simulink library "outp"  (R2021b)
(part 3 of 10)

  bus_selector16/53 -> outpmodule/942(VVMC_ADASLDWSta_enum)  "<VVMC_ADASLDWSta_enum>"
  outpmodule/395(VOUTP_OBC4PreDTC_raw32) -> bus_creator/395
  outpmodule/345(VOUTP_HMIKey7FuncSta_enum) -> bus_creator/345
  outpmodule/919(VOUTP_LKATOIFault_flg) -> bus_creator/919
  outpmodule/560(VOUTP_DCDCEnaReq_flg) -> bus_creator/560
  outpmodule/917(VOUTP_ADASLKASta_enum) -> bus_creator/917
  bus_selector4/61 -> outpmodule/420(VDDM_DiagFRTSDTC_raw32)  "<VDDM_DiagFRTSDTC_raw32>"
  outpmodule/576(VOUTP_PwrDownReq_enum) -> bus_creator/576
  outpmodule/621(VOUTP_Change1_cnt) -> bus_creator/621
  outpmodule/622(VOUTP_Change2_cnt) -> bus_creator/622
  bus_selector2/83 -> outpmodule/86(VAPM_RRPulseCountTimeOut_flg)  "<VAPM_RRPulseCountTimeOut_flg>"
  outpmodule/624(VOUTP_SHA1_cnt) -> bus_creator/624
  outpmodule/187(VOUTP_DrDoorSW_flg) -> bus_creator/187
  outpmodule/990(VOUTP_CAASActive_flg) -> bus_creator/990
  outpmodule/623(VOUTP_Dash2_cnt) -> bus_creator/623
  outpmodule/620(VOUTP_Dash1_cnt) -> bus_creator/620
  outpmodule/783(VOUTP_RRP20_raw8) -> bus_creator/783
  outpmodule/618(VOUTP_Country2_cnt) -> bus_creator/618
  outpmodule/234(VOUTP_AmbLightBrightness3_enum) -> bus_creator/234
  outpmodule/509(VOUTP_CAN1BusErrorDTC_raw32) -> bus_creator/509
  bus_selector2/34 -> outpmodule/37(VAPM_USSStaFLR_flg)  "<VAPM_USSStaFLR_flg>"
  outpmodule/619(VOUTP_Variation_cnt) -> bus_creator/619
  outpmodule/176(VOUTP_RAPSErrWarnSta_enum) -> bus_creator/176
  outpmodule/617(VOUTP_Country1_cnt) -> bus_creator/617
  outpmodule/616(VOUTP_Patch2_cnt) -> bus_creator/616
  outpmodule/985(VOUTP_APSReq_enum) -> bus_creator/985
  outpmodule/613(VOUTP_Minor1_cnt) -> bus_creator/613
  bus_selector3/164 -> outpmodule/342(VBCM_HMIKey4FuncSta_enum)  "<VBCM_HMIKey4FuncSta_enum>"
  outpmodule/767(VOUTP_LFSensorMode_flg) -> bus_creator/767
  outpmodule/538(VOUTP_FDCDKCAllowSleep_flg) -> bus_creator/538
  outpmodule/615(VOUTP_Patch1_cnt) -> bus_creator/615
  bus_selector16/66 -> outpmodule/955(VVMC_ADASLaneModeR_enum)  "<VVMC_ADASLaneModeR_enum>"
  outpmodule/614(VOUTP_Minor2_cnt) -> bus_creator/614
  outpmodule/349(VOUTP_PasWdwReqAP_enum) -> bus_creator/349
  outpmodule/552(VOUTP_ActiveWU_flg) -> bus_creator/552
  outpmodule/611(VOUTP_Major1_cnt) -> bus_creator/611
  outpmodule/612(VOUTP_Major2_cnt) -> bus_creator/612
  outpmodule/335(VOUTP_AutoLockSta_flg) -> bus_creator/335
  BTHC_outputs/1 -> bus_selector11/1
  outpmodule/609(VOUTP_ECU1_cnt) -> bus_creator/609
  outpmodule/324(VOUTP_PTGUserHeight7_cnt) -> bus_creator/324
  bus_selector3/21 -> outpmodule/199(VBCM_DimmerEN_flg)  "<VBCM_DimmerEN_flg>"
  outpmodule/321(VOUTP_PTGUserHeight3_cnt) -> bus_creator/321
  outpmodule/981(VOUTP_APSActive_flg) -> bus_creator/981
  outpmodule/530(VOUTP_DKeyWelcomeSta_enum) -> bus_creator/530
  outpmodule/608(VOUTP_CarModel3_cnt) -> bus_creator/608
  outpmodule/166(VOUTP_DKCPDkeyAreaRAPSSta_enum) -> bus_creator/166
  outpmodule/606(VOUTP_CarModel1_cnt) -> bus_creator/606
  bus_selector12/75 -> outpmodule/804(VTPM_WriteChkRFID_raw)  "<VTPM_WriteChkRFID_raw>"
  bus_selector11/36 -> outpmodule/681(VTHC_sigAmbAirT_C)  "<VTHC_sigAmbAirT_C>"
  outpmodule/129(VOUTP_EPBExtReleaseAvail_flg) -> bus_creator/129
  outpmodule/607(VOUTP_CarModel2_cnt) -> bus_creator/607
  outpmodule/219(VOUTP_TrunkRel_flg) -> bus_creator/219
  outpmodule/603(VOUTP_HWVer1_cnt) -> bus_creator/603
  outpmodule/604(VOUTP_HWVer2_cnt) -> bus_creator/604
  bus_selector4/96 -> outpmodule/455(VDDM_ISAMalfuncDetDTC_raw32)  "<VDDM_ISAMalfuncDetDTC_raw32>"
  bus_selector3/39 -> outpmodule/217(VBCM_RoomLampH_flg)  "<VBCM_RoomLampH_flg>"
  outpmodule/434(VOUTP_RLRUSSDTC_raw32) -> bus_creator/434
  outpmodule/364(VOUTP_C3BMS1CSDTC_raw32) -> bus_creator/364
  outpmodule/602(VOUTP_PwrReqRAPSAvail_flg) -> bus_creator/602
  outpmodule/749(VOUTP_RRWheelDebug_flg) -> bus_creator/749
  outpmodule/556(VOUTP_PowerDownState_enum) -> bus_creator/556
  outpmodule/601(VOUTP_OTAPwrReqStdChkSta_enum) -> bus_creator/601
  outpmodule/863(VOUTP_RrUdcMax_V) -> bus_creator/863
  bus_selector11/9 -> outpmodule/654(VTHC_FDTWVCmd_pct)  "<VTHC_FDTWVCmd_pct>"
  outpmodule/932(VOUTP_ACCJerkLowerLimit_mps3) -> bus_creator/932
  outpmodule/599(VOUTP_PwrReq_OTA_enum) -> bus_creator/599
  bus_selector10/22 -> outpmodule/624(VSYS_SHA1_cnt)  "<VSYS_SHA1_cnt>"
  outpmodule/600(VOUTP_OTAPwrReqOFFChkSta_enum) -> bus_creator/600
  bus_selector6/15 -> outpmodule/535(VDKC_ParkingModeCmd_enum)  "<VDKC_ParkingModeCmd_enum>"
  outpmodule/597(VOUTP_PwrStaTOSta_enum) -> bus_creator/597
  outpmodule/390(VOUTP_MidLvSaChkDTC_raw32) -> bus_creator/390
  outpmodule/351(VOUTP_PsRWdwReqAP_enum) -> bus_creator/351
  outpmodule/459(VOUTP_MCUR1CSErrDTC_raw32) -> bus_creator/459
  outpmodule/133(VOUTP_EPBErrSta_enum) -> bus_creator/133
  outpmodule/596(VOUTP_CtrlDrPwrStbA2_flg) -> bus_creator/596
  outpmodule/329(VOUTP_TimeGapLevelSta_enum) -> bus_creator/329
  outpmodule/595(VOUTP_HWResetSta_enum) -> bus_creator/595
  outpmodule/377(VOUTP_Lv3ErrDTC_raw32) -> bus_creator/377
  outpmodule/593(VOUTP_CtrlFrBMSCCUCIR_flg) -> bus_creator/593
  outpmodule/801(VOUTP_LRPindi_enum) -> bus_creator/801
  bus_selector13/34 -> outpmodule/860(VTQD_RrIdcMin_A)  "<VTQD_RrIdcMin_A>"
  outpmodule/675(VOUTP_sigSetTempZon1St_C) -> bus_creator/675
  outpmodule/491(VOUTP_LimpHomeActTmp_flg) -> bus_creator/491
  bus_selector13/37 -> outpmodule/863(VTQD_RrUdcMax_V)  "<VTQD_RrUdcMax_V>"
  bus_selector10/30 -> outpmodule/632(VSYS_NvWriteReqRisingEdge_flg)  "<VSYS_NvWriteReqRisingEdge_flg>"
  outpmodule/782(VOUTP_LRP20_raw8) -> bus_creator/782
  outpmodule/646(VOUTP_FDCompCmd_rpm) -> bus_creator/646
  bus_selector16/102 -> outpmodule/991(VVMC_ExtraMSACtrlSta_enum)  "<VVMC_ExtraMSACtrlSta_enum>"
  outpmodule/373(VOUTP_C1ABM1CSDTC_raw32) -> bus_creator/373
  bus_selector13/35 -> outpmodule/861(VTQD_RrIdcMax_A)  "<VTQD_RrIdcMax_A>"
  bus_selector16/56 -> outpmodule/945(VVMC_ForceLowBeam_enum)  "<VVMC_ForceLowBeam_enum>"
  bus_selector13/36 -> outpmodule/862(VTQD_RrUdcMin_V)  "<VTQD_RrUdcMin_V>"
  outpmodule/226(VOUTP_AmbLightBreath1_enum) -> bus_creator/226
  outpmodule/378(VOUTP_Lv4ErrDTC_raw32) -> bus_creator/378
  bus_selector13/45 -> outpmodule/871(VTQD_ExtDoorAllow_flg)  "<VTQD_ExtDoorAllow_flg>"
  outpmodule/819(VOUTP_FlashS4ID_raw) -> bus_creator/819
  bus_selector2/91 -> outpmodule/94(VAPM_SASAngleTimeOut_flg)  "<VAPM_SASAngleTimeOut_flg>"
  bus_selector13/42 -> outpmodule/868(VTQD_DriveProtEn_flg)  "<VTQD_DriveProtEn_flg>"
  outpmodule/487(VOUTP_5vAPS1PwrErrDTC_raw32) -> bus_creator/487
  outpmodule/960(VOUTP_ADASLFCHandsOffWarning_enum) -> bus_creator/960
  bus_selector2/51 -> outpmodule/54(VAPM_RRRawWhlSpeedTimeOut_flg)  "<VAPM_RRRawWhlSpeedTimeOut_flg>"
  outpmodule/587(VOUTP_PMMAllowECUSleep_flg) -> bus_creator/587
  bus_selector13/39 -> outpmodule/865(VTQD_ExtShftAllow_flg)  "<VTQD_ExtShftAllow_flg>"
  outpmodule/951(VOUTP_LKAHODDisplayWarning_flg) -> bus_creator/951
  outpmodule/320(VOUTP_PTGUserHeight2_cnt) -> bus_creator/320
  bus_selector13/38 -> outpmodule/864(VTQD_ReBrakeLPReq_flg)  "<VTQD_ReBrakeLPReq_flg>"
  outpmodule/958(VOUTP_ADASLDWMute_flg) -> bus_creator/958
  BSYS_outputs/1 -> bus_selector10/1
  outpmodule/547(VOUTP_ErrorState_enum) -> bus_creator/547
  outpmodule/591(VOUTP_CtrlFrPwrStbA1P_flg) -> bus_creator/591
  outpmodule/203(VOUTP_RrFogLamp_flg) -> bus_creator/203
  bus_selector2/96 -> outpmodule/99(VAPM_SASCAL_flg)  "<VAPM_SASCAL_flg>"
  outpmodule/464(VOUTP_ESC1RCErrDTC_raw32) -> bus_creator/464
  bus_selector2/22 -> outpmodule/25(VAPM_PASARCL_enum)  "<VAPM_PASARCL_enum>"
  bus_selector2/19 -> outpmodule/22(VAPM_PASARMR_enum)  "<VAPM_PASARMR_enum>"
  outpmodule/999(VOUTP_FDCVMCAPSAngleTarget_deg) -> bus_creator/999
  bus_selector4/91 -> outpmodule/450(VDDM_CCUSigErrDetDTC_raw32)  "<VDDM_CCUSigErrDetDTC_raw32>"
  outpmodule/539(VOUTP_DISCTurn_flg) -> bus_creator/539
  outpmodule/169(VOUTP_CAASVMCReqA_flg) -> bus_creator/169
  bus_selector2/17 -> outpmodule/20(VAPM_APSDFLL_cm)  "<VAPM_APSDFLL_cm>"
  outpmodule/577(VOUTP_LowSOCWarn_enum) -> bus_creator/577
  bus_selector2/18 -> outpmodule/21(VAPM_PASAFCL_enum)  "<VAPM_PASAFCL_enum>"
  outpmodule/665(VOUTP_BatteryMode_enum) -> bus_creator/665
  outpmodule/1003(VOUTP_FDCVMCMaxAngCtrlOutTqLim_Nm) -> bus_creator/1003
  bus_selector2/15 -> outpmodule/18(VAPM_APSDRLL_cm)  "<VAPM_APSDRLL_cm>"
  bus_selector4/127 -> outpmodule/486(VDDM_C1EPAS2LCDTC_raw32)  "<VDDM_C1EPAS2LCDTC_raw32>"
  outpmodule/791(VOUTP_ID2messageALTU_raw8) -> bus_creator/791
  outpmodule/131(VOUTP_EPBExtApplyAvail_flg) -> bus_creator/131
  bus_selector2/10 -> outpmodule/13(VAPM_PASDFMR_cm)  "<VAPM_PASDFMR_cm>"
  bus_selector2/14 -> outpmodule/17(VAPM_APSDRLR_cm)  "<VAPM_APSDRLR_cm>"
  bus_selector2/13 -> outpmodule/16(VAPM_PASDFCL_cm)  "<VAPM_PASDFCL_cm>"
  bus_selector2/68 -> outpmodule/71(VAPM_LFPulseCountV_flg)  "<VAPM_LFPulseCountV_flg>"
  bus_selector2/89 -> outpmodule/92(VAPM_EPSAOIControlTimeOut_flg)  "<VAPM_EPSAOIControlTimeOut_flg>"
  outpmodule/947(VOUTP_ADASWarningMsg_enum) -> bus_creator/947
  bus_selector13/40 -> outpmodule/866(VTQD_CreepON_flg)  "<VTQD_CreepON_flg>"
  outpmodule/374(VOUTP_C1ABM1LCDTC_raw32) -> bus_creator/374
  bus_selector2/87 -> outpmodule/90(VAPM_DriIntendTimeOut_flg)  "<VAPM_DriIntendTimeOut_flg>"
  bus_selector2/81 -> outpmodule/84(VAPM_LRPulseCountTimeOut_flg)  "<VAPM_LRPulseCountTimeOut_flg>"
  bus_selector2/35 -> outpmodule/38(VAPM_USSStaFLL_flg)  "<VAPM_USSStaFLL_flg>"
  bus_selector2/8 -> outpmodule/11(VAPM_PASDRCR_cm)  "<VAPM_PASDRCR_cm>"
  bus_selector2/97 -> outpmodule/100(VAPM_SASCALTimeOut_flg)  "<VAPM_SASCALTimeOut_flg>"
  outpmodule/467(VOUTP_ESC5CSErrDTC_raw32) -> bus_creator/467
  outpmodule/598(VOUTP_Sched_ChgTOSta_enum) -> bus_creator/598
  bus_selector16/41 -> outpmodule/930(VVMC_ACCJerkUpperLimit_mps3)  "<VVMC_ACCJerkUpperLimit_mps3>"
  bus_selector2/9 -> outpmodule/12(VAPM_PASDRCL_cm)  "<VAPM_PASDRCL_cm>"
  bus_selector4/55 -> outpmodule/414(VDDM_ESC7NoComDTC_raw32)  "<VDDM_ESC7NoComDTC_raw32>"
  bus_selector2/6 -> outpmodule/9(VAPM_PASDRMR_cm)  "<VAPM_PASDRMR_cm>"
  bus_selector9/33 -> outpmodule/587(VPMM_PMMAllowECUSleep_flg)  "<VPMM_PMMAllowECUSleep_flg>"
  bus_selector4/116 -> outpmodule/475(VDDM_RFPressIndiDTC_raw32)  "<VDDM_RFPressIndiDTC_raw32>"
  bus_selector2/31 -> outpmodule/34(VAPM_USSStaRCL_flg)  "<VAPM_USSStaRCL_flg>"
  bus_selector13/32 -> outpmodule/858(VTQD_FrUdcMin_V)  "<VTQD_FrUdcMin_V>"
  outpmodule/772(VOUTP_S2ID_raw32) -> bus_creator/772
  bus_selector2/7 -> outpmodule/10(VAPM_PASDRML_cm)  "<VAPM_PASDRML_cm>"
  bus_selector2/5 -> outpmodule/8(VAPM_ChrgPlugSta_enum)  "<VAPM_ChrgPlugSta_enum>"
  outpmodule/455(VOUTP_ISAMalfuncDetDTC_raw32) -> bus_creator/455
  outpmodule/209(VOUTP_RBSD_flg) -> bus_creator/209
  bus_selector2/3 -> outpmodule/6(VAPM_FSOffSw_enum)  "<VAPM_FSOffSw_enum>"
  bus_selector2/2 -> outpmodule/5(VAPM_VehSpeedTimeOut_flg)  "<VAPM_VehSpeedTimeOut_flg>"
  outpmodule/642(VOUTP_DrivingMode_cnt) -> bus_creator/642
  outpmodule/380(VOUTP_BrkSWNoBacDTC_raw32) -> bus_creator/380
  outpmodule/49(VOUTP_RFRawWhlSpeed_kph) -> bus_creator/49
  bus_selector2/1 -> outpmodule/4(VAPM_VehSpeed_kph)  "<VAPM_VehSpeed_kph>"
  outpmodule/32(VOUTP_USSStaRLL_flg) -> bus_creator/32
  bus_selector2/4 -> outpmodule/7(VAPM_FSOffSwTimeOut_flg)  "<VAPM_FSOffSwTimeOut_flg>"
  outpmodule/143(VOUTP_AVMErrSTA_flg) -> bus_creator/143
  bus_selector4/115 -> outpmodule/474(VDDM_LFPressIndiDTC_raw32)  "<VDDM_LFPressIndiDTC_raw32>"
  outpmodule/563(VOUTP_HVSysReadyToCharge_enum) -> bus_creator/563
  bus_selector2/124 -> outpmodule/127(VAPM_ESCAPSSta_enum)  "<VAPM_ESCAPSSta_enum>"
  bus_selector2/29 -> outpmodule/32(VAPM_USSStaRLL_flg)  "<VAPM_USSStaRLL_flg>"
  outpmodule/972(VOUTP_ADASAEBSta_enum) -> bus_creator/972
  bus_selector4/121 -> outpmodule/480(VDDM_LRWheelTmpHighDTC_raw32)  "<VDDM_LRWheelTmpHighDTC_raw32>"
  outpmodule/796(VOUTP_TPMSStorge_flg) -> bus_creator/796
  outpmodule/440(VOUTP_FCM3CSErrDTC_raw32) -> bus_creator/440
  bus_selector2/28 -> outpmodule/31(VAPM_USSStaRLR_flg)  "<VAPM_USSStaRLR_flg>"
  outpmodule/871(VOUTP_ExtDoorAllow_flg) -> bus_creator/871
  bus_selector2/151 -> outpmodule/154(VAPM_TCSActiveTimeOut_flg)  "<VAPM_TCSActiveTimeOut_flg>"
  bus_selector16/25 -> outpmodule/914(VVMC_FeatArbitrFinal_enum)  "<VVMC_FeatArbitrFinal_enum>"
  bus_selector11/60 -> outpmodule/705(VTHC_FDCTHCDrEVentYSta_enum)  "<VTHC_FDCTHCDrEVentYSta_enum>"
  bus_selector2/27 -> outpmodule/30(VAPM_USSStaRML_flg)  "<VAPM_USSStaRML_flg>"
  outpmodule/139(VOUTP_AVMparkingexcute_enum) -> bus_creator/139
  bus_selector2/25 -> outpmodule/28(VAPM_PASAFCR_enum)  "<VAPM_PASAFCR_enum>"
  outpmodule/331(VOUTP_ACCLevelMem34_enum) -> bus_creator/331
  bus_selector3/59 -> outpmodule/237(VBCM_AmbLightBrightness6_enum)  "<VBCM_AmbLightBrightness6_enum>"
  outpmodule/882(VOUTP_RrTMTqReq_Nm) -> bus_creator/882
  bus_selector2/26 -> outpmodule/29(VAPM_USSStaRMR_flg)  "<VAPM_USSStaRMR_flg>"
  outpmodule/952(VOUTP_LKAHODSoundWarning_flg) -> bus_creator/952
  bus_selector12/86 -> outpmodule/815(VTPM_Prepresstempvalid_enum)  "<VTPM_Prepresstempvalid_enum>"
  bus_selector16/20 -> outpmodule/909(VVMC_ISOAccLimit_mps2)  "<VVMC_ISOAccLimit_mps2>"
  bus_selector2/131 -> outpmodule/134(VAPM_EPBErrStaTimeOut_flg)  "<VAPM_EPBErrStaTimeOut_flg>"
  bus_selector10/21 -> outpmodule/623(VSYS_Dash2_cnt)  "<VSYS_Dash2_cnt>"
  bus_selector2/24 -> outpmodule/27(VAPM_PASAFML_enum)  "<VAPM_PASAFML_enum>"
  outpmodule/190(VOUTP_RRDoorSW_flg) -> bus_creator/190
  outpmodule/458(VOUTP_MCUF1CSErrDTC_raw32) -> bus_creator/458
  bus_selector2/23 -> outpmodule/26(VAPM_PASAFMR_enum)  "<VAPM_PASAFMR_enum>"
  bus_selector11/79 -> outpmodule/724(VTHC_FDCFGSIONCmd_flg)  "<VTHC_FDCFGSIONCmd_flg>"
  bus_selector3/143 -> outpmodule/321(VBCM_PTGUserHeight3_cnt)  "<VBCM_PTGUserHeight3_cnt>"
  outpmodule/173(VOUTP_RAPSBCMLamp_enum) -> bus_creator/173
  outpmodule/312(VOUTP_WalkOutLkENFunSta_flg) -> bus_creator/312
  outpmodule/896(VOUTP_VMCCCCtrlAvail_flg) -> bus_creator/896
  bus_selector3/2 -> outpmodule/180(VBCM_TailgateRemote_enum)  "<VBCM_TailgateRemote_enum>"
  bus_selector2/12 -> outpmodule/15(VAPM_PASDFCR_cm)  "<VAPM_PASDFCR_cm>"
  bus_selector3/1 -> outpmodule/179(VBCM_AntitheftSta_enum)  "<VBCM_AntitheftSta_enum>"
  outpmodule/484(VOUTP_LRSensorFailDTC_raw32) -> bus_creator/484
  bus_selector3/163 -> outpmodule/341(VBCM_HMIKey3FuncSta_enum)  "<VBCM_HMIKey3FuncSta_enum>"
  bus_selector2/74 -> outpmodule/77(VAPM_RRPulseCountV_flg)  "<VAPM_RRPulseCountV_flg>"
  outpmodule/934(VOUTP_ADASVehSpdLim_raw32) -> bus_creator/934
  bus_selector2/73 -> outpmodule/76(VAPM_LRPulseCountVTimeOut_flg)  "<VAPM_LRPulseCountVTimeOut_flg>"
  bus_selector4/144 -> outpmodule/503(VDDM_VCUFRDoorSta_flg)  "<VDDM_VCUFRDoorSta_flg>"
  bus_selector6/17 -> outpmodule/537(VDKC_KeyTypeSta_enum)  "<VDKC_KeyTypeSta_enum>"
  bus_selector2/72 -> outpmodule/75(VAPM_LRPulseCountV_flg)  "<VAPM_LRPulseCountV_flg>"
  bus_selector11/53 -> outpmodule/698(VTHC_FDCTHCAirIntZ3Sta_enum)  "<VTHC_FDCTHCAirIntZ3Sta_enum>"
  outpmodule/895(VOUTP_VMCACCCtrlAvail_flg) -> bus_creator/895
  outpmodule/476(VOUTP_LRPressIndiDTC_raw32) -> bus_creator/476
  outpmodule/142(VOUTP_AVMParkingmodeTimeOut_flg) -> bus_creator/142
  bus_selector2/84 -> outpmodule/87(VAPM_ShifterHandleCmd_enum)  "<VAPM_ShifterHandleCmd_enum>"
  bus_selector11/16 -> outpmodule/661(VTHC_FDFrLeAPTCHeatPwrCmd_W)  "<VTHC_FDFrLeAPTCHeatPwrCmd_W>"
  outpmodule/69(VOUTP_RRWhlRotDir_enum) -> bus_creator/69
  outpmodule/68(VOUTP_LRWhlRotDirTimeOut_flg) -> bus_creator/68
  bus_selector16/64 -> outpmodule/953(VVMC_ADASLFCSta_enum)  "<VVMC_ADASLFCSta_enum>"
  bus_selector11/57 -> outpmodule/702(VTHC_FDCTHCCLEVentZSta_enum)  "<VTHC_FDCTHCCLEVentZSta_enum>"
  bus_selector2/11 -> outpmodule/14(VAPM_PASDFML_cm)  "<VAPM_PASDFML_cm>"
  bus_selector8/6 -> outpmodule/548(VNMM_NodeID_enum)  "<VNMM_NodeID_enum>"
  outpmodule/66(VOUTP_RFWhlRotDirTimeOut_flg) -> bus_creator/66
  outpmodule/472(VOUTP_LRBatwarnDTC_raw32) -> bus_creator/472
  bus_selector3/95 -> outpmodule/273(VBCM_AmbWelENFlash_enum)  "<VBCM_AmbWelENFlash_enum>"
  outpmodule/67(VOUTP_LRWhlRotDir_enum) -> bus_creator/67
  bus_selector12/43 -> outpmodule/772(VTPM_S2ID_raw32)  "<VTPM_S2ID_raw32>"
  bus_selector4/78 -> outpmodule/437(VDDM_FCM2CSErrDTC_raw32)  "<VDDM_FCM2CSErrDTC_raw32>"
  bus_selector6/12 -> outpmodule/532(VDKC_KeyAreaSPTGSta_enum)  "<VDKC_KeyAreaSPTGSta_enum>"
  outpmodule/65(VOUTP_RFWhlRotDir_enum) -> bus_creator/65
  bus_selector12/79 -> outpmodule/808(VTPM_WriteChkfinRFID_raw)  "<VTPM_WriteChkfinRFID_raw>"
  outpmodule/64(VOUTP_LFWhlRotDirTimeOut_flg) -> bus_creator/64
  outpmodule/751(VOUTP_TPMSCaliButtAllow_flg) -> bus_creator/751
  outpmodule/63(VOUTP_LFWhlRotDir_enum) -> bus_creator/63
  outpmodule/542(VOUTP_DISCButtSta_flg) -> bus_creator/542
  outpmodule/265(VOUTP_AmbODAEN_flg) -> bus_creator/265
  outpmodule/182(VOUTP_AllDoorSW_flg) -> bus_creator/182
  outpmodule/61(VOUTP_RRRawWhlSpeedV_flg) -> bus_creator/61
  outpmodule/520(VOUTP_EAPS2NRM_pct) -> bus_creator/520
  outpmodule/976(VOUTP_ACCPedalOvrd_flg) -> bus_creator/976
  outpmodule/62(VOUTP_RRRawWhlSpeedVTimeOut_flg) -> bus_creator/62
  bus_selector12/93 -> outpmodule/822(VTPM_TPMSTLCmd_flg)  "<VTPM_TPMSTLCmd_flg>"
  outpmodule/361(VOUTP_C3BMS6CSDTC_raw32) -> bus_creator/361
  outpmodule/389(VOUTP_HiLvSaChkDTC_raw32) -> bus_creator/389
  bus_selector3/64 -> outpmodule/242(VBCM_AmbLightColor5_enum)  "<VBCM_AmbLightColor5_enum>"
  outpmodule/120(VOUTP_MCPressureVTimeOut_flg) -> bus_creator/120
  outpmodule/387(VOUTP_BMSRdyDTC_raw32) -> bus_creator/387
  outpmodule/118(VOUTP_LongAccelVTimeOut_flg) -> bus_creator/118
  outpmodule/117(VOUTP_LongAccelV_flg) -> bus_creator/117
  bus_selector11/31 -> outpmodule/676(VTHC_sigSetTempZon2St_C)  "<VTHC_sigSetTempZon2St_C>"
  outpmodule/116(VOUTP_LatAccelVTimeOut_flg) -> bus_creator/116
  outpmodule/327(VOUTP_PTGOpenHeight57_enum) -> bus_creator/327
  outpmodule/873(VOUTP_SaveRegenMode_enum) -> bus_creator/873
  bus_selector13/2 -> outpmodule/828(VTQD_TqSourceFr_enum)  "<VTQD_TqSourceFr_enum>"
  outpmodule/115(VOUTP_LatAccelV_flg) -> bus_creator/115
  outpmodule/241(VOUTP_AmbLightColor4_enum) -> bus_creator/241
  outpmodule/762(VOUTP_LRWheelPSW_raw8) -> bus_creator/762
  outpmodule/114(VOUTP_YawRateVTimeOut_flg) -> bus_creator/114
  bus_selector4/119 -> outpmodule/478(VDDM_LFWheelTmpHighDTC_raw32)  "<VDDM_LFWheelTmpHighDTC_raw32>"
  outpmodule/549(VOUTP_PNI_flg) -> bus_creator/549
  bus_selector12/36 -> outpmodule/765(VTPM_CWheelTips_enum)  "<VTPM_CWheelTips_enum>"
  outpmodule/993(VOUTP_CalibratedAccY_G) -> bus_creator/993
  outpmodule/111(VOUTP_MCPressure_bar) -> bus_creator/111
  outpmodule/251(VOUTP_MirrorFlodPos_flg) -> bus_creator/251
  outpmodule/432(VOUTP_FLRUSSDTC_raw32) -> bus_creator/432
  bus_selector3/50 -> outpmodule/228(VBCM_AmbLightBreath3_enum)  "<VBCM_AmbLightBreath3_enum>"
  outpmodule/356(VOUTP_WinLROpenedSta_pct) -> bus_creator/356
  bus_selector3/68 -> outpmodule/246(VBCM_APSOpenPTG_flg)  "<VBCM_APSOpenPTG_flg>"
  outpmodule/967(VOUTP_FCMACCmode_enum) -> bus_creator/967
  outpmodule/113(VOUTP_YawRateV_flg) -> bus_creator/113
  bus_selector13/4 -> outpmodule/830(VTQD_FrEDUAvailBrkRgnTq_Nm)  "<VTQD_FrEDUAvailBrkRgnTq_Nm>"
  outpmodule/718(VOUTP_FDCFGSAirIntSta_enum) -> bus_creator/718
  outpmodule/337(VOUTP_AutoUnlockSta_flg) -> bus_creator/337
  bus_selector3/56 -> outpmodule/234(VBCM_AmbLightBrightness3_enum)  "<VBCM_AmbLightBrightness3_enum>"
  outpmodule/959(VOUTP_ADASFCWMute_flg) -> bus_creator/959
  bus_selector9/14 -> outpmodule/568(VPMM_FrMCUEnaReq_flg)  "<VPMM_FrMCUEnaReq_flg>"
  outpmodule/711(VOUTP_FDCTHCCREVentYSta_enum) -> bus_creator/711
  bus_selector2/150 -> outpmodule/153(VAPM_TCSActive_flg)  "<VAPM_TCSActive_flg>"
  outpmodule/112(VOUTP_MCPressureTimeOut_flg) -> bus_creator/112
  outpmodule/20(VOUTP_APSDFLL_cm) -> bus_creator/20
  outpmodule/109(VOUTP_LongAccel_Gps) -> bus_creator/109
  outpmodule/528(VOUTP_KeyAreaLockUnlock_enum) -> bus_creator/528
  bus_selector4/56 -> outpmodule/415(VDDM_ESC1NoComDTC_raw32)  "<VDDM_ESC1NoComDTC_raw32>"
  bus_selector10/36 -> outpmodule/638(VSYS_CurrentNmState_enum)  "<VSYS_CurrentNmState_enum>"
  bus_selector16/21 -> outpmodule/910(VVMC_ISODecLimit_mps2)  "<VVMC_ISODecLimit_mps2>"
  bus_selector4/123 -> outpmodule/482(VDDM_LFSensorFailDTC_raw32)  "<VDDM_LFSensorFailDTC_raw32>"
  bus_selector3/127 -> outpmodule/305(VBCM_HBeamADB_flg)  "<VBCM_HBeamADB_flg>"
  outpmodule/110(VOUTP_LongAccelTimeOut_flg) -> bus_creator/110
  bus_selector11/71 -> outpmodule/716(VTHC_PsVentEN_flg)  "<VTHC_PsVentEN_flg>"
  outpmodule/444(VOUTP_FCM5CSErrDTC_raw32) -> bus_creator/444
  outpmodule/108(VOUTP_LatAccelTimeOut_flg) -> bus_creator/108
  bus_selector2/153 -> outpmodule/156(VAPM_DriverSeatBeltCmdTimeOut_flg)  "<VAPM_DriverSeatBeltCmdTimeOut_flg>"
  outpmodule/106(VOUTP_YawRateTimeOut_flg) -> bus_creator/106
  outpmodule/195(VOUTP_CTDCtrl_enum) -> bus_creator/195
  bus_selector12/12 -> outpmodule/741(VTPM_RRWheelTemp_C)  "<VTPM_RRWheelTemp_C>"
  outpmodule/679(VOUTP_sigClntTHvBattIn_C) -> bus_creator/679
  outpmodule/107(VOUTP_LatAccel_Gps) -> bus_creator/107
  outpmodule/723(VOUTP_FDCFGSIONSWSta_flg) -> bus_creator/723
  bus_selector4/48 -> outpmodule/407(VDDM_VehMalfunLevel_enum)  "<VDDM_VehMalfunLevel_enum>"
  outpmodule/104(VOUTP_GRADETimeOut_flg) -> bus_creator/104
  outpmodule/105(VOUTP_YawRate_degps) -> bus_creator/105
  outpmodule/101(VOUTP_SASV_flg) -> bus_creator/101
  bus_selector11/63 -> outpmodule/708(VTHC_FDCTHCCLVentENSta_flg)  "<VTHC_FDCTHCCLVentENSta_flg>"
  outpmodule/102(VOUTP_SASVTimeOut_flg) -> bus_creator/102
  bus_selector3/122 -> outpmodule/300(VBCM_TurnSwTimeSetSta123_enum)  "<VBCM_TurnSwTimeSetSta123_enum>"
  outpmodule/103(VOUTP_GRADE_Deg) -> bus_creator/103
  outpmodule/569(VOUTP_RrMCUEnaReq_flg) -> bus_creator/569
  outpmodule/301(VOUTP_TurnSwTimeSetSta457_enum) -> bus_creator/301
  outpmodule/754(VOUTP_LRPressIndi_enum) -> bus_creator/754
  outpmodule/100(VOUTP_SASCALTimeOut_flg) -> bus_creator/100
  outpmodule/96(VOUTP_SASSpeedTimeOut_flg) -> bus_creator/96
  bus_selector2/30 -> outpmodule/33(VAPM_USSStaRCR_flg)  "<VAPM_USSStaRCR_flg>"
  outpmodule/180(VOUTP_TailgateRemote_enum) -> bus_creator/180
  outpmodule/98(VOUTP_SASSpeedValidTimeOut_flg) -> bus_creator/98
  bus_selector16/17 -> outpmodule/906(VVMC_SafetyCtrl_flg)  "<VVMC_SafetyCtrl_flg>"
  outpmodule/95(VOUTP_SASSpeed_degps) -> bus_creator/95
  bus_selector3/66 -> outpmodule/244(VBCM_LampPwr_flg)  "<VBCM_LampPwr_flg>"
  outpmodule/851(VOUTP_RgnAbnorSta_flg) -> bus_creator/851
  outpmodule/88(VOUTP_ShifterHandleCmdTimeOut_flg) -> bus_creator/88
  bus_selector2/75 -> outpmodule/78(VAPM_RRPulseCountVTimeOut_flg)  "<VAPM_RRPulseCountVTimeOut_flg>"
  outpmodule/511(VOUTP_CAN3BusErrorDTC_raw32) -> bus_creator/511
  outpmodule/978(VOUTP_CCCtrlSta_enum) -> bus_creator/978
  outpmodule/94(VOUTP_SASAngleTimeOut_flg) -> bus_creator/94
  outpmodule/610(VOUTP_ECU2_cnt) -> bus_creator/610
  outpmodule/87(VOUTP_ShifterHandleCmd_enum) -> bus_creator/87
  bus_selector3/89 -> outpmodule/267(VBCM_AmbBrightSta_enum)  "<VBCM_AmbBrightSta_enum>"
  bus_selector2/125 -> outpmodule/128(VAPM_ESCAPSStaTimeOut_flg)  "<VAPM_ESCAPSStaTimeOut_flg>"
  outpmodule/443(VOUTP_FCM5NoComDTC_raw32) -> bus_creator/443
  bus_selector12/64 -> outpmodule/793(VTPM_ID4messageALTU_raw8)  "<VTPM_ID4messageALTU_raw8>"
  bus_selector16/87 -> outpmodule/976(VVMC_ACCPedalOvrd_flg)  "<VVMC_ACCPedalOvrd_flg>"
  outpmodule/84(VOUTP_LRPulseCountTimeOut_flg) -> bus_creator/84
  bus_selector11/39 -> outpmodule/684(VTHC_FDRecyAutoCmd_enum)  "<VTHC_FDRecyAutoCmd_enum>"
  bus_selector11/72 -> outpmodule/717(VTHC_CRVentEN_flg)  "<VTHC_CRVentEN_flg>"
  bus_selector2/37 -> outpmodule/40(VAPM_USSStaFCL_flg)  "<VAPM_USSStaFCL_flg>"
  outpmodule/352(VOUTP_CLWinLockDrSta_flg) -> bus_creator/352
  outpmodule/85(VOUTP_RRPulseCount_enum) -> bus_creator/85
  outpmodule/318(VOUTP_UserHeightSet_cnt) -> bus_creator/318
  outpmodule/80(VOUTP_LFPulseCountTimeOut_flg) -> bus_creator/80
  bus_selector3/130 -> outpmodule/308(VBCM_RmLpModeENMem_enum)  "<VBCM_RmLpModeENMem_enum>"
  bus_selector2/20 -> outpmodule/23(VAPM_PASARML_enum)  "<VAPM_PASARML_enum>"
  outpmodule/79(VOUTP_LFPulseCount_enum) -> bus_creator/79
  outpmodule/470(VOUTP_LFBatwarnDTC_raw32) -> bus_creator/470
  outpmodule/181(VOUTP_HornCtrl_flg) -> bus_creator/181
  bus_selector3/38 -> outpmodule/216(VBCM_RrDefog_flg)  "<VBCM_RrDefog_flg>"
  bus_selector16/100 -> outpmodule/989(VVMC_CAASCtrlAvail_flg)  "<VVMC_CAASCtrlAvail_flg>"
  bus_selector9/32 -> outpmodule/586(VPMM_FDADC12VDetAvg_mV)  "<VPMM_FDADC12VDetAvg_mV>"
  bus_selector4/97 -> outpmodule/456(VDDM_MCUF1RCErrDTC_raw32)  "<VDDM_MCUF1RCErrDTC_raw32>"
  outpmodule/76(VOUTP_LRPulseCountVTimeOut_flg) -> bus_creator/76
  outpmodule/987(VOUTP_CCMSASpdWar_flg) -> bus_creator/987
  outpmodule/437(VOUTP_FCM2CSErrDTC_raw32) -> bus_creator/437
  bus_selector4/27 -> outpmodule/386(VDDM_HVRlyCloDTC_raw32)  "<VDDM_HVRlyCloDTC_raw32>"
  bus_selector2/38 -> outpmodule/41(VAPM_Chime_enum)  "<VAPM_Chime_enum>"
  outpmodule/73(VOUTP_RFPulseCountV_flg) -> bus_creator/73
  outpmodule/346(VOUTP_HMIKey8FuncSta_enum) -> bus_creator/346
  outpmodule/70(VOUTP_RRWhlRotDirTimeOut_flg) -> bus_creator/70
  bus_selector4/126 -> outpmodule/485(VDDM_RRSensorFailDTC_raw32)  "<VDDM_RRSensorFailDTC_raw32>"
  bus_selector2/67 -> outpmodule/70(VAPM_RRWhlRotDirTimeOut_flg)  "<VAPM_RRWhlRotDirTimeOut_flg>"
  outpmodule/93(VOUTP_SASAngle_Deg) -> bus_creator/93
  bus_selector13/16 -> outpmodule/842(VTQD_RrEDUActTq_Nm)  "<VTQD_RrEDUActTq_Nm>"
  outpmodule/354(VOUTP_WinLFOpenedSta_pct) -> bus_creator/354
  bus_selector2/159 -> outpmodule/162(VAPM_APSAngleTarget_Deg)  "<VAPM_APSAngleTarget_Deg>"
  bus_selector4/22 -> outpmodule/381(VDDM_KeyAuthDTC_raw32)  "<VDDM_KeyAuthDTC_raw32>"
  outpmodule/962(VOUTP_LVDAMuteSta_enum) -> bus_creator/962
  outpmodule/625(VOUTP_SHA2_cnt) -> bus_creator/625
  outpmodule/156(VOUTP_DriverSeatBeltCmdTimeOut_flg) -> bus_creator/156
  bus_selector9/37 -> outpmodule/591(VPMM_CtrlFrPwrStbA1P_flg)  "<VPMM_CtrlFrPwrStbA1P_flg>"
  outpmodule/535(VOUTP_ParkingModeCmd_enum) -> bus_creator/535
  outpmodule/695(VOUTP_fdefog_flg) -> bus_creator/695
  bus_selector3/121 -> outpmodule/299(VBCM_OutMode_enum)  "<VBCM_OutMode_enum>"
  outpmodule/706(VOUTP_FDCTHCDrVentENSta_flg) -> bus_creator/706
  bus_selector4/155 -> outpmodule/514(VDDM_CAN6BusErrorDTC_raw32)  "<VDDM_CAN6BusErrorDTC_raw32>"
  bus_selector16/115 -> outpmodule/1004(VVMC_FDCVMCDrInpTqBstGn_pct)  "<VVMC_FDCVMCDrInpTqBstGn_pct>"
  bus_selector16/113 -> outpmodule/1002(VVMC_FDCVMCDrInpTqBstAct_flg)  "<VVMC_FDCVMCDrInpTqBstAct_flg>"
  outpmodule/168(VOUTP_PUIDLowPower_flg) -> bus_creator/168
  bus_selector2/163 -> outpmodule/166(VAPM_DKCPDkeyAreaRAPSSta_enum)  "<VAPM_DKCPDkeyAreaRAPSSta_enum>"
  outpmodule/1002(VOUTP_FDCVMCDrInpTqBstAct_flg) -> bus_creator/1002
  outpmodule/92(VOUTP_EPSAOIControlTimeOut_flg) -> bus_creator/92
  bus_selector4/82 -> outpmodule/441(VDDM_FCM4NoComDTC_raw32)  "<VDDM_FCM4NoComDTC_raw32>"
  bus_selector4/92 -> outpmodule/451(VDDM_ACCAccelCmdErrDetDTC_raw32)  "<VDDM_ACCAccelCmdErrDetDTC_raw32>"
  outpmodule/449(VOUTP_RrMCUSigErrDetDTC_raw32) -> bus_creator/449
  bus_selector16/111 -> outpmodule/1000(VVMC_FDCVMCAPSRqEPSCtrl_flg)  "<VVMC_FDCVMCAPSRqEPSCtrl_flg>"
  bus_selector16/112 -> outpmodule/1001(VVMC_FDCVMCAngCtrlTqWtGn_pct)  "<VVMC_FDCVMCAngCtrlTqWtGn_pct>"
  outpmodule/8(VOUTP_ChrgPlugSta_enum) -> bus_creator/8
  bus_selector9/16 -> outpmodule/570(VPMM_DrivetrainSelect_enum)  "<VPMM_DrivetrainSelect_enum>"
  outpmodule/164(VOUTP_APSRqEPASCtrl_flg) -> bus_creator/164
  bus_selector16/114 -> outpmodule/1003(VVMC_FDCVMCMaxAngCtrlOutTqLim_Nm)  "<VVMC_FDCVMCMaxAngCtrlOutTqLim_Nm>"
  bus_selector3/107 -> outpmodule/285(VBCM_AmbBrightnessSta2_enum)  "<VBCM_AmbBrightnessSta2_enum>"
  bus_selector13/41 -> outpmodule/867(VTQD_EquivAccPedalSWSta_flg)  "<VTQD_EquivAccPedalSWSta_flg>"
  bus_selector11/38 -> outpmodule/683(VTHC_ACSubMode_enum)  "<VTHC_ACSubMode_enum>"
  bus_selector16/106 -> outpmodule/995(VVMC_CalibratedGyroX_Dps)  "<VVMC_CalibratedGyroX_Dps>"
  outpmodule/322(VOUTP_PTGUserHeight4_cnt) -> bus_creator/322
  bus_selector16/6 -> outpmodule/895(VVMC_VMCACCCtrlAvail_flg)  "<VVMC_VMCACCCtrlAvail_flg>"
  outpmodule/435(VOUTP_FCM2NoComDTC_raw32) -> bus_creator/435
  outpmodule/99(VOUTP_SASCAL_flg) -> bus_creator/99
  bus_selector16/104 -> outpmodule/993(VVMC_CalibratedAccY_G)  "<VVMC_CalibratedAccY_G>"
  bus_selector16/107 -> outpmodule/996(VVMC_CalibratedGyroY_Dps)  "<VVMC_CalibratedGyroY_Dps>"
  bus_selector4/152 -> outpmodule/511(VDDM_CAN3BusErrorDTC_raw32)  "<VDDM_CAN3BusErrorDTC_raw32>"
  outpmodule/83(VOUTP_LRPulseCount_enum) -> bus_creator/83
  outpmodule/246(VOUTP_APSOpenPTG_flg) -> bus_creator/246
  outpmodule/454(VOUTP_MSAMalfuncDetDTC_raw32) -> bus_creator/454
  bus_selector4/7 -> outpmodule/366(VDDM_C3CCU1RCDTC_raw32)  "<VDDM_C3CCU1RCDTC_raw32>"
  outpmodule/89(VOUTP_DriIntend_enum) -> bus_creator/89
  bus_selector11/46 -> outpmodule/691(VTHC_CCUSyncSts_flg)  "<VTHC_CCUSyncSts_flg>"
  bus_selector16/108 -> outpmodule/997(VVMC_CalibratedGyroZ_Dps)  "<VVMC_CalibratedGyroZ_Dps>"
  bus_selector3/140 -> outpmodule/318(VBCM_UserHeightSet_cnt)  "<VBCM_UserHeightSet_cnt>"
  bus_selector4/134 -> outpmodule/493(VDDM_EngagePFail_flg)  "<VDDM_EngagePFail_flg>"
  outpmodule/145(VOUTP_IVIStatus_flg) -> bus_creator/145
  bus_selector16/103 -> outpmodule/992(VVMC_CalibratedAccX_G)  "<VVMC_CalibratedAccX_G>"
  outpmodule/163(VOUTP_APSVRqEPASCtrl_flg) -> bus_creator/163
  bus_selector4/132 -> outpmodule/491(VDDM_LimpHomeActTmp_flg)  "<VDDM_LimpHomeActTmp_flg>"
  outpmodule/311(VOUTP_WalkInUnLkENFunSta_flg) -> bus_creator/311
  outpmodule/674(VOUTP_sigRecircSt_flg) -> bus_creator/674
  outpmodule/71(VOUTP_LFPulseCountV_flg) -> bus_creator/71
  outpmodule/557(VOUTP_PowerUpFault_enum) -> bus_creator/557
  outpmodule/91(VOUTP_EPSAOIControl_enum) -> bus_creator/91
  bus_selector16/105 -> outpmodule/994(VVMC_CalibratedAccZ_G)  "<VVMC_CalibratedAccZ_G>"
  bus_selector2/120 -> outpmodule/123(VAPM_BrkSwV_flg)  "<VAPM_BrkSwV_flg>"
  bus_selector2/59 -> outpmodule/62(VAPM_RRRawWhlSpeedVTimeOut_flg)  "<VAPM_RRRawWhlSpeedVTimeOut_flg>"
  outpmodule/496(VOUTP_VCURAPSErrLv3_flg) -> bus_creator/496
  bus_selector16/48 -> outpmodule/937(VVMC_ADASForceIdle_flg)  "<VVMC_ADASForceIdle_flg>"
  outpmodule/572(VOUTP_PwrStaSelect_enum) -> bus_creator/572
  bus_selector3/115 -> outpmodule/293(VBCM_FWipSwSta_enum)  "<VBCM_FWipSwSta_enum>"
  outpmodule/151(VOUTP_ABSActive_flg) -> bus_creator/151
  outpmodule/984(VOUTP_APSDecReq_mps2) -> bus_creator/984
  outpmodule/77(VOUTP_RRPulseCountV_flg) -> bus_creator/77
  outpmodule/193(VOUTP_RrChargingDoorCtrl_enum) -> bus_creator/193
  bus_selector12/96 -> outpmodule/825(VTPM_ModelVersion_raw)  "<VTPM_ModelVersion_raw>"
  outpmodule/461(VOUTP_Shifter1CSErrDTC_raw32) -> bus_creator/461
  outpmodule/279(VOUTP_AmbColorSta2_enum) -> bus_creator/279
  outpmodule/150(VOUTP_IVIScreenTimeOut_flg) -> bus_creator/150
  outpmodule/227(VOUTP_AmbLightBreath2_enum) -> bus_creator/227
  outpmodule/149(VOUTP_IVIScreen_enum) -> bus_creator/149
  outpmodule/81(VOUTP_RFPulseCount_enum) -> bus_creator/81
  bus_selector11/18 -> outpmodule/663(VTHC_FDRrAPTCHeatPwrCmd_W)  "<VTHC_FDRrAPTCHeatPwrCmd_W>"
  outpmodule/97(VOUTP_SASSpeedValid_flg) -> bus_creator/97
  bus_selector2/16 -> outpmodule/19(VAPM_APSDFLR_cm)  "<VAPM_APSDFLR_cm>"
  outpmodule/660(VOUTP_FDEWP3Cmd_enum) -> bus_creator/660
  outpmodule/78(VOUTP_RRPulseCountVTimeOut_flg) -> bus_creator/78
  bus_selector4/11 -> outpmodule/370(VDDM_C3CCU2CSDTC_raw32)  "<VDDM_C3CCU2CSDTC_raw32>"
  bus_selector2/56 -> outpmodule/59(VAPM_LRRawWhlSpeedV_flg)  "<VAPM_LRRawWhlSpeedV_flg>"
  outpmodule/383(VOUTP_HVB4PreDTC_raw32) -> bus_creator/383
  outpmodule/833(VOUTP_ShiftGearPosn_enum) -> bus_creator/833
  outpmodule/148(VOUTP_CAASSwTimeOut_flg) -> bus_creator/148
  bus_selector16/10 -> outpmodule/899(VVMC_FeatReqSpd_kph)  "<VVMC_FeatReqSpd_kph>"
  outpmodule/213(VOUTP_BCMBuzzerReq_flg) -> bus_creator/213
  outpmodule/147(VOUTP_CAASSw_enum) -> bus_creator/147
  bus_selector16/110 -> outpmodule/999(VVMC_FDCVMCAPSAngleTarget_deg)  "<VVMC_FDCVMCAPSAngleTarget_deg>"
  outpmodule/146(VOUTP_IVIStatusTimeOut_flg) -> bus_creator/146
  outpmodule/330(VOUTP_ACCLevelMem12_enum) -> bus_creator/330
  bus_selector3/120 -> outpmodule/298(VBCM_SPTGENFunMem_enum)  "<VBCM_SPTGENFunMem_enum>"
  outpmodule/698(VOUTP_FDCTHCAirIntZ3Sta_enum) -> bus_creator/698
  outpmodule/263(VOUTP_AmbLinkDriSta_flg) -> bus_creator/263
  outpmodule/90(VOUTP_DriIntendTimeOut_flg) -> bus_creator/90
  bus_selector2/21 -> outpmodule/24(VAPM_PASARCR_enum)  "<VAPM_PASARCR_enum>"
  outpmodule/605(VOUTP_HWVer3_cnt) -> bus_creator/605
  bus_selector3/117 -> outpmodule/295(VBCM_TurnSwSta_enum)  "<VBCM_TurnSwSta_enum>"
  outpmodule/75(VOUTP_LRPulseCountV_flg) -> bus_creator/75
  outpmodule/524(VOUTP_KeyMissSta_flg) -> bus_creator/524
  bus_selector13/7 -> outpmodule/833(VTQD_ShiftGearPosn_enum)  "<VTQD_ShiftGearPosn_enum>"
  bus_selector3/113 -> outpmodule/291(VBCM_DimSwSta_flg)  "<VBCM_DimSwSta_flg>"
  bus_selector3/41 -> outpmodule/219(VBCM_TrunkRel_flg)  "<VBCM_TrunkRel_flg>"
  outpmodule/903(VOUTP_RearWhlSlipRatioCtrl_flg) -> bus_creator/903
  outpmodule/74(VOUTP_RFPulseCountVTimeOut_flg) -> bus_creator/74
  outpmodule/333(VOUTP_LRightStaCmd_flg) -> bus_creator/333
  bus_selector3/119 -> outpmodule/297(VBCM_SPTGENFun_flg)  "<VBCM_SPTGENFun_flg>"
  outpmodule/72(VOUTP_LFPulseCountVTimeOut_flg) -> bus_creator/72
  bus_selector12/60 -> outpmodule/789(VTPM_S4WheelDebugALTU_pct)  "<VTPM_S4WheelDebugALTU_pct>"
  bus_selector16/68 -> outpmodule/957(VVMC_ADASISASta_enum)  "<VVMC_ADASISASta_enum>"
  bus_selector4/143 -> outpmodule/502(VDDM_VCUFLDoorSta_flg)  "<VDDM_VCUFLDoorSta_flg>"
  bus_selector3/26 -> outpmodule/204(VBCM_BrakeLamp_flg)  "<VBCM_BrakeLamp_flg>"
  outpmodule/522(VOUTP_DKCAuthSta_enum) -> bus_creator/522
  bus_selector3/116 -> outpmodule/294(VBCM_FWasSwSta_enum)  "<VBCM_FWasSwSta_enum>"
  outpmodule/586(VOUTP_FDADC12VDetAvg_mV) -> bus_creator/586
  bus_selector6/5 -> outpmodule/525(VDKC_KeyModeSta_enum)  "<VDKC_KeyModeSta_enum>"
  outpmodule/224(VOUTP_WasherCtrl_enum) -> bus_creator/224
  bus_selector16/109 -> outpmodule/998(VVMC_FDCVMCAPSVRqEPSCtrl_flg)  "<VVMC_FDCVMCAPSVRqEPSCtrl_flg>"
  outpmodule/534(VOUTP_DkeyAreaRAPSSta_enum) -> bus_creator/534
  outpmodule/86(VOUTP_RRPulseCountTimeOut_flg) -> bus_creator/86
  bus_selector12/15 -> outpmodule/744(VTPM_LRSensorFail_flg)  "<VTPM_LRSensorFail_flg>"
  BVMC_outputs/1 -> bus_selector16/1
  bus_selector4/28 -> outpmodule/387(VDDM_BMSRdyDTC_raw32)  "<VDDM_BMSRdyDTC_raw32>"
  bus_selector16/8 -> outpmodule/897(VVMC_VMCMSACtrlAvail_flg)  "<VVMC_VMCMSACtrlAvail_flg>"
  outpmodule/367(VOUTP_C3CCU1CSDTC_raw32) -> bus_creator/367
  outpmodule/594(VOUTP_CtrlFrEDUINVERTER_flg) -> bus_creator/594
  bus_selector3/112 -> outpmodule/290(VBCM_HazardIND_flg)  "<VBCM_HazardIND_flg>"
  outpmodule/729(VOUTP_EWPBUflag3_flg) -> bus_creator/729
  outpmodule/204(VOUTP_BrakeLamp_flg) -> bus_creator/204
  outpmodule/82(VOUTP_RFPulseCountTimeOut_flg) -> bus_creator/82
  outpmodule/501(VOUTP_VCUBrkSWSta_enum) -> bus_creator/501
  outpmodule/471(VOUTP_RFBatwarnDTC_raw32) -> bus_creator/471
  bus_selector3/111 -> outpmodule/289(VBCM_AmbBrightnessSta7_enum)  "<VBCM_AmbBrightnessSta7_enum>"
  outpmodule/527(VOUTP_KeyAreaPS_enum) -> bus_creator/527
  bus_selector6/3 -> outpmodule/523(VDKC_TimeSNDKCFbk_cnt)  "<VDKC_TimeSNDKCFbk_cnt>"
  bus_selector16/37 -> outpmodule/926(VVMC_ADASACCSta_enum)  "<VVMC_ADASACCSta_enum>"
